simulink model "UnifiedControlPathTrackingDriver"  (R2026b)
settings: Solver=FixedStepDiscrete  StopTime=0.1  FixedStep=UnifiedControlSampleTime
undefined symbols (not defined in the file): EnableEnergyManagement, EnableRegen, EnableTC, EnableTV, UnifiedControlEnableEnergyManagement, UnifiedControlEnableRegen, UnifiedControlEnableTC, UnifiedControlEnableTV
settings Model: DataDictionary=VehicleData.sldd  Creator=Xu Dingyi  LastModifiedBy=29358

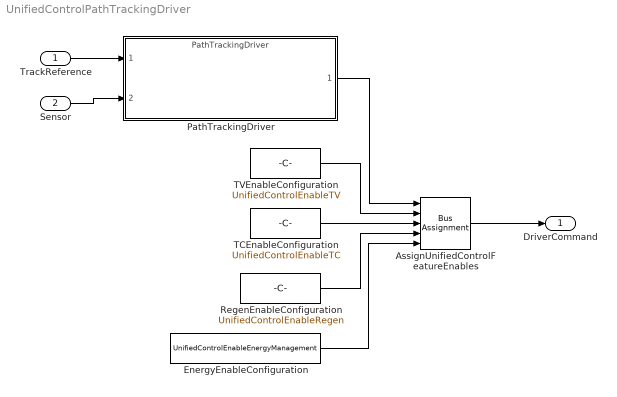
== system UnifiedControlPathTrackingDriver ==
  TrackReference : Inport  OutDataTypeStr=Bus: TrackReferenceBus
  Sensor : Inport  Port=2  OutDataTypeStr=Bus: SensorBus
  AssignUnifiedControlFeatureEnables : BusAssignment  AssignedSignals=EnableTV,EnableTC,EnableRegen,EnableEnergyManagement
  EnergyEnableConfiguration : Constant  Value=UnifiedControlEnableEnergyManagement  OutDataTypeStr=boolean
  PathTrackingDriver : ModelReference  ModelNameDialog=PathTrackingDriver  ModelReferenceVersion=2.0
  RegenEnableConfiguration : Constant  Value=UnifiedControlEnableRegen  OutDataTypeStr=boolean
  TCEnableConfiguration : Constant  Value=UnifiedControlEnableTC  OutDataTypeStr=boolean
  TVEnableConfiguration : Constant  Value=UnifiedControlEnableTV  OutDataTypeStr=boolean
  DriverCommand : Outport  OutDataTypeStr=Bus: DriverCommandBus
  wires:
  Sensor/1 -> PathTrackingDriver/2
  TrackReference/1 -> PathTrackingDriver/1
  PathTrackingDriver/1 -> AssignUnifiedControlFeatureEnables/1
  TCEnableConfiguration/1 -> AssignUnifiedControlFeatureEnables/3
  TVEnableConfiguration/1 -> AssignUnifiedControlFeatureEnables/2
  EnergyEnableConfiguration/1 -> AssignUnifiedControlFeatureEnables/5
  RegenEnableConfiguration/1 -> AssignUnifiedControlFeatureEnables/4
  AssignUnifiedControlFeatureEnables/1 -> DriverCommand/1
